simulink model "PedalSensor"  (R2024b)
settings: Solver=FixedStepAuto  StartTime=0.0  StopTime=1  RelTol=1e-3
libraries: SignalEditorBlockLib x1
settings Model: Creator=bew  LastModifiedBy=bew
settings OptimizationCC: DefaultParameterBehavior=Inlined  EnhancedBackFolding=on  PassReuseOutputArgsAs=Individual arguments  ZeroExternalMemoryAtStartup=off  ZeroInternalMemoryAtStartup=off  OptimizeBlockOrder=speed  DifferentSizesBufferReuse=on  OptimizationCustomize=off  EfficientTunableParamExpr=on
settings DebuggingCC: ParameterTunabilityLossMsg=error
settings SFSimCC: MATLABDynamicMemAlloc=off
settings RTWCC: Description=Embedded Coder  SystemTargetFile=ert.tlc  TemplateMakefile=ert_default_tmf
settings CodeAppCC: ForceParamTrailComments=on  IgnoreCustomStorageClasses=off  OperatorAnnotations=on  SimulinkDataObjDesc=on  SFDataObjDesc=on  InsertBlockDesc=on
settings ERTTargetCC: TargetLangStandard=C99 (ISO)  GenerateSampleERTMain=on  ERTCustomFileTemplate=example_file_process.tlc

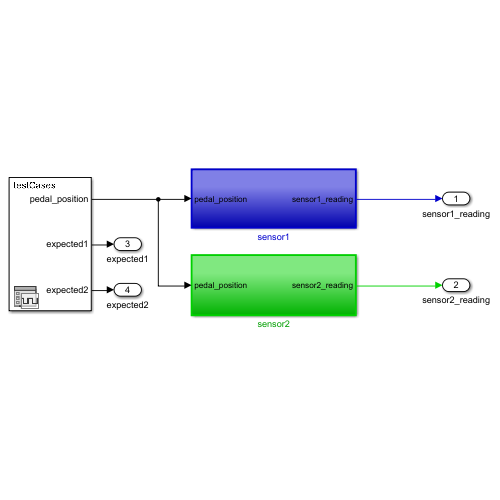
[thumbnail: Simulink's stored preview of the top-level diagram]
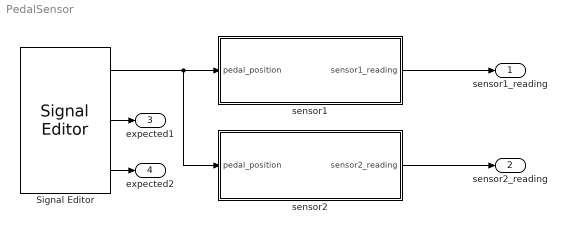
== system PedalSensor ==
  Signal Editor : SignalEditorBlockLib/Signal Editor  FileName=TestSignal.mat  ActiveScenario=testCases  ActiveSignal=pedal_position  IsBus=off  OutputBusObjectStr=Bus: BusObject  SampleTime=0  Interpolate=off  ZeroCross=off  OutputAfterFinalValue=Setting to zero  Unit=inherit  PreserveSignalName=on  ApplySigPropsToAllScenarios=on  ApplySigPropsToAllSignals=off
  sensor1 : Subsystem  TreatAsAtomicUnit=on
  sensor2 : Subsystem  TreatAsAtomicUnit=on
  sensor1_reading : Outport
  sensor2_reading : Outport  Port=2
  expected1 : Outport  Port=3
  expected2 : Outport  Port=4
  wires:
  sensor2/1(sensor2_reading) -> sensor2_reading/1
  Signal Editor/1 -> sensor2/1(pedal_position), sensor1/1(pedal_position)
  sensor1/1(sensor1_reading) -> sensor1_reading/1
  Signal Editor/2 -> expected1/1
  Signal Editor/3 -> expected2/1

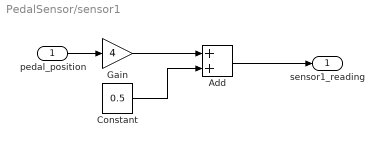
== system PedalSensor/sensor1 ==
  pedal_position : Inport
  Add : Sum
  Constant : Constant  Value=0.5
  Gain : Gain  Gain=4
  sensor1_reading : Outport
  wires:
  Constant/1 -> Add/2
  Gain/1 -> Add/1
  pedal_position/1 -> Gain/1
  Add/1 -> sensor1_reading/1

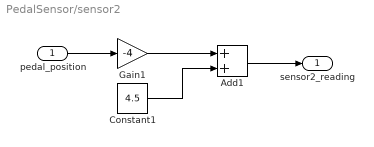
== system PedalSensor/sensor2 ==
  pedal_position : Inport
  Add1 : Sum
  Constant1 : Constant  Value=4.5
  Gain1 : Gain  Gain=-4
  sensor2_reading : Outport
  wires:
  Constant1/1 -> Add1/2
  Add1/1 -> sensor2_reading/1
  Gain1/1 -> Add1/1
  pedal_position/1 -> Gain1/1
